simulink model "Pendulum"  (R2024b)
settings: Solver=ode45  StartTime=0.0  StopTime=20  MaxStep=1e-2  RelTol=1e-3  EnableMultiTasking=on
InitFcn:
  | g = 9.81; %gravitational constant
  | 
  | %% S-function
  | % showVR = 0;
  | % CartBlocking = 0;
  | % CartHard = 0;
  | % phi0 = 0; %initial conditions
values from neighbouring files (symbols this model uses):
  A_down = double(subs(A_sym, [X; u], [X_down; u_eq]))    [linearization.m]    (also in my_pendulum.m)
  B_down = double(subs(B_sym, [X; u], [X_down; u_eq]))    [linearization.m]    (also in my_pendulum.m)
  C = [0 1 0 0 ... (first row only)    [linearization.m]    (also in my_pendulum.m)
  D = [0; 0]    [linearization.m]    (also in my_pendulum.m)
  Kp = 10.2    [my_pendulum.m]
libraries: vrlib x4, slpidlib x1
CloseFcn:
  | vrclose all;
  | clear figureVR worldVR;
settings Model: Creator=H  LastModifiedBy=jx2004
settings SolverCC: AlgebraicLoopSolver=TrustRegion
settings DataIOCC: LimitDataPoints=on  SaveFormat=Array  SignalLoggingSaveFormat=ModelDataLogs  ReturnWorkspaceOutputs=off
settings OptimizationCC: ExpressionDepthLimit=2147483647  InitFltsAndDblsToZero=on  LifeSpan=inf
settings DebuggingCC: SaveWithParameterizedLinksMsg=none  UnderspecifiedInitializationDetection=Classic  MergeDetectMultiDrivingBlocksExec=none  SignalResolutionControl=TryResolveAllWithWarning  SolverPrmCheckMsg=warning  FcnCallInpInsideContextMsg=warning  UnconnectedInputMsg=warning  UnconnectedOutputMsg=warning  UnconnectedLineMsg=warning  StateNameClashWarn=warning  SFUnexpectedBacktrackingDiag=warning  SFNoUnconditionalDefaultTransitionDiag=warning  SFExecutionAtInitializationDiag=none  ArithmeticOperatorsInVariantConditions=warning
settings HardwareCC: ProdBitPerPointer=32  ProdBitPerSizeT=32  ProdBitPerPtrDiffT=32  ProdLargestAtomicFloat=None  ProdIntDivRoundTo=Undefined  ProdEndianess=Unspecified  ProdWordSize=32  ProdHWDeviceType=32-bit Generic
settings ModelReferenceCC: PropagateSignalLabelsOutOfModel=off
settings SFSimCC: SimUseLocalCustomCode=off  CustomCodeUndefinedFunction=UseInterfaceOnly
settings RTWCC: RTWUseLocalCustomCode=off  GPUComputeCapability=3.5
settings CodeAppCC: StateflowObjectComments=on
settings GRTTargetCC: TargetFcnLib=ansi_tfl_tmw.mat  TargetLangStandard=C89/C90 (ANSI)  CombineOutputUpdateFcns=off  GRTInterface=on
settings ConfigComp: CovMetricSettings=dw  CovSaveCumulativeToWorkspaceVar=on  CovSaveSingleToWorkspaceVar=on  CovExternalEMLEnable=off

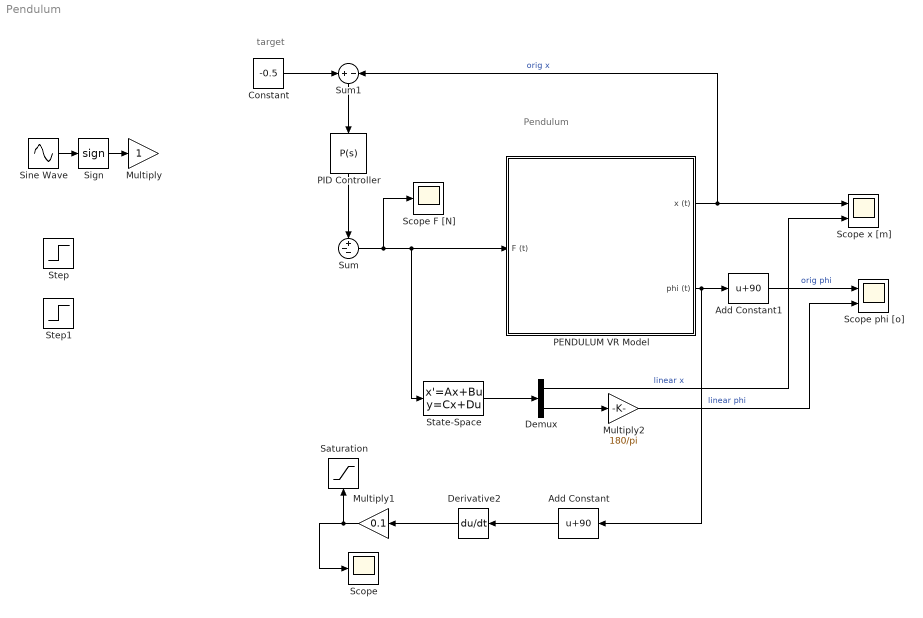
== system Pendulum ==
  note: target
  note: Pendulum
  Add Constant : Bias  Bias=90  SaturateOnIntegerOverflow=off
  Add Constant1 : Bias  Bias=90  SaturateOnIntegerOverflow=off
  Constant : Constant  Value=-0.5
  Demux : Demux  Outputs=2
  Derivative2 : Derivative
  Multiply : Gain
  Multiply1 : Gain  Gain=0.1
  Multiply2 : Gain  Gain=180/pi
  PENDULUM VR Model : Subsystem  mask(Pendulum){showVR=on, phi0=-90, y0=0, brake=off, rail_bound=off}
      mask prompts: showVR "Show Virtual World?"; phi0 "Initial angle of the pendulum   phi(0) [deg] (from horizontal plane)"; y0 "Initial position of the cart x0 [m] (rightwise from the center)"; brake "Cart brake"; rail_bound "Obey rail boundaries"
      mask help: Pendulum - Virtual Reality
      mask init:
      | clear figureVR worldVR;
      | showVR = 1;
      mask Help:
      | Pendulum - Virtual Reality. <br><br>
      | 
      | This is a model of the inverted pendulum on a cart, which consit of a beam and a cart. The beam is connected with the cart by a pivot. The input of this system is mechanical force applied on the cart, outputs are the angle of the beam and the position of the cart.   <br><br>
      | 
      | 
      | In the mask of the model, it can be set:
      | <ul>
      | <li>Initial angle of the pendulum</li>
      | </ul><br><br>
      | 
      | 
      | Copyright: 2007,   Jan Vana, Jirka Roubal, Petr Husek.
      mask Callback showVR:
      | if strcmp('off',get_param(gcb,'showVR'))
      |     vrclose all;
      | else
      |     if exist('figureVR')==0
      |         figureVR = vrfigure;
      |     end
      |     if exist('worldVR')==0
      |         worldVR = vrworld('Pendulum_VR.WRL');
      |     end
      | 	if isvalid(figureVR)==0
      |         open(worldVR);
      |         figureVR = vrfigure(worldVR,[650 80 550 350]);
      | 	end
      | end
      mask Display:
      | image(imread('Pendulum_Image.jpg'))
      | port_label ('input',1,'F')
      | port_label ('output',1,'x')
      | port_label ('output',2,'phi')
  PID Controller : slpidlib/PID Controller  Controller=P  Form=Parallel  TimeDomain=Continuous-time  UseExternalTs=off  SampleTime=-1  IntegratorMethod=Forward Euler  FilterMethod=Forward Euler  ControllerParametersSource=internal  P=Kp  I=1  UseKiTs=off  D=1  UseExternalDerivativeSource=off  N=100  UseFilter=on  TunerSelectOption=Transfer Function Based (PID Tuner App)  InitialConditionSource=internal  InitialConditionForIntegrator=0  InitialConditionForFilter=0  DifferentiatorICPrevScaledInput=0  ExternalReset=none  TrackingMode=off  Kt=1  LimitOutput=off  SatLimitsSource=internal  UpperSaturationLimit=inf  LowerSaturationLimit=-inf  LinearizeAsGain=on  AntiWindupMode=none  Kb=1  LimitIntegrator=off  UpperIntegratorSaturationLimit=inf  LowerIntegratorSaturationLimit=-inf  POutMin=[]  POutMax=[]  IOutMin=[]  IOutMax=[]  DOutMin=[]  DOutMax=[]  NOutMin=[]  NOutMax=[]  SumOutMin=[]  SumOutMax=[]  SaturationOutMin=[]  SaturationOutMax=[]  PParamMin=[]  PParamMax=[]  IParamMin=[]  IParamMax=[]  DParamMin=[]  DParamMax=[]  NParamMin=[]  NParamMax=[]  KbParamMin=[]  KbParamMax=[]  KtParamMin=[]  KtParamMax=[]  KbOutMin=[]  KbOutMax=[]  KtOutMin=[]  KtOutMax=[]  IntegratorOutMin=[]  IntegratorOutMax=[]  FilterOutMin=[]  FilterOutMax=[]  SumI1OutMin=[]  SumI1OutMax=[]  SumI2OutMin=[]  SumI2OutMax=[]  SumI3OutMin=[]  SumI3OutMax=[]  SumI4OutMin=[]  SumI4OutMax=[]  SumDOutMin=[]  SumDOutMax=[]  DifferentiatorOutMin=[]  DifferentiatorOutMax=[]  FilterDiffOutCoefMin=[]  FilterDiffOutCoefMax=[]  ReciprocalOutMin=[]  ReciprocalOutMax=[]  SumDenOutMin=[]  SumDenOutMax=[]  SumNumOutMin=[]  SumNumOutMax=[]  DivideOutMin=[]  DivideOutMax=[]  UdiffTsProdOutMin=[]  UdiffTsProdOutMax=[]  NTsProdOutMin=[]  NTsProdOutMax=[]  UintegralTsProdOutMin=[]  UintegralTsProdOutMax=[]  UngainTsProdOutMin=[]  UngainTsProdOutMax=[]  ClampingZeroOutDataTypeStr=Inherit: Inherit via back propagation  ClampingZeroOutMin=[]  ClampingZeroOutMax=[]  FilterDenConstantOutDataTypeStr=Inherit: Inherit via back propagation  FilterDenConstantOutMin=[]  FilterDenConstantOutMax=[]  PCopyOutDataTypeStr=Inherit: Inherit via back propagation  PCopyOutMin=[]  PCopyOutMax=[]  NCopyOutDataTypeStr=Inherit: Inherit via back propagation  NCopyOutMin=[]  NCopyOutMax=[]  IntegratorContinuousStateAttributes=''  IntegratorStateMustResolveToSignalObject=off  IntegratorRTWStateStorageClass=Auto  FilterContinuousStateAttributes=''  FilterStateMustResolveToSignalObject=off  FilterRTWStateStorageClass=Auto  ParallelPVariant=InternalParameters  IdealPVariant=Disabled  IVariant=Disabled  DVariant=Disabled  IntegratorVariant=Disabled  SatVariant=Disabled  AWVariant=Disabled  PCopyVariant=Disabled  TRVariant=Disabled  FdbkBlocksVariant=Forward  IdealPFdbkVariant=Disabled  SatFdbkVariant=Disabled  DerivativeFilterVariant=Disabled  NVariant=Disabled  NCopyVariant=Disabled_SignalSpec  FilterICVariant=Disabled  IntegratorICVariant=Disabled  ExternalResetVariant=Disabled  TRSumVariant=Passthrough  SumFdbkVariant=Disabled  SumVariant=Passthrough_P  TsampFilterVariant=InternalTs  TsampNgainVariant=Passthrough  TsampIntegralVariant=Disabled_SignalSpec  ExternalSaturationOutDataTypeStr=Inherit: Same as second input  DerivativeSourceVariant=Disabled  PreIntVariant=InternalPreInt
  Saturation : Saturate  UpperLimit=10  LowerLimit=-10  LinearizeAsGain=off  ZeroCross=off
  Scope : Scope
  Scope phi [o] : Scope  NumInputPorts=2
  Scope x [m] : Scope  NumInputPorts=2
  Scope F [N] : Scope
  Sign : Signum
  Sine Wave : Sin  Frequency=1.2  SampleTime=0
  State-Space : StateSpace  A=A_down  B=B_down  C=C  D=D  InitialCondition=[0; 0; 0; 0]
  Step : Step  Time=0  After=5  SampleTime=0
  Step1 : Step  Time=2  After=5  SampleTime=0
  Sum : Sum  Inputs=+--
  Sum1 : Sum  Inputs=+-
  wires:
  Sum/1 -> Scope F [N]/1, State-Space/1, PENDULUM VR Model/1(F (t))
  PENDULUM VR Model/2(phi (t)) -> Add Constant1/1, Add Constant/1
  Sine Wave/1 -> Sign/1
  Sign/1 -> Multiply/1
  Multiply1/1 -> Scope/1, Saturation/1
  Derivative2/1 -> Multiply1/1
  Add Constant/1 -> Derivative2/1
  State-Space/1 -> Demux/1
  Demux/1 -> Scope x [m]/2  "linear x"
  Demux/2 -> Multiply2/1
  Add Constant1/1 -> Scope phi [o]/1  "orig phi"
  Multiply2/1 -> Scope phi [o]/2  "linear phi"
  PENDULUM VR Model/1(x (t)) -> Sum1/2, Scope x [m]/1  "orig x"
  Constant/1 -> Sum1/1
  Sum1/1 -> PID Controller/1
  PID Controller/1 -> Sum/1

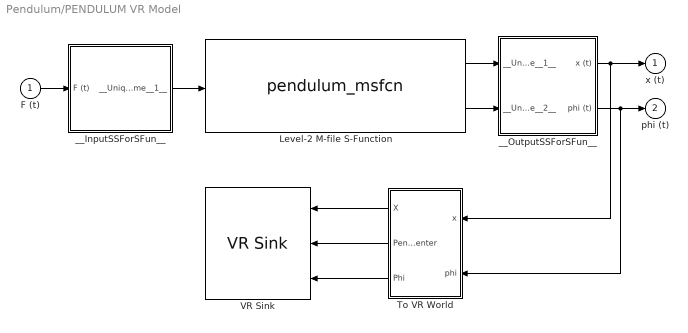
== system Pendulum/PENDULUM VR Model ==
  F (t) : Inport
  Level-2 M-file S-Function : M-S-Function  FunctionName=pendulum_msfcn  Parameters=y0, phi0, rail_bound, brake
  To VR World : Subsystem
  VR Sink : vrlib/VR Sink  InstantiateOnLoad=on  SampleTime=0.1  ViewEnable=on  RemoteChange=off  RemoteView=on  FieldsWritten=cart.translation.3.1.double#pendulum.center.3.1.double#pendulum.rotation.4.1.double  WorldFileName=Pendulum_VR.WRL  AutoView=off  VideoDimensions=[]  AllowVariableSize=off
  __InputSSForSFun__ : Subsystem
  __OutputSSForSFun__ : Subsystem
  x (t) : Outport  OutDataTypeStr=double  PortDimensions=1  SampleTime=[-1 0]
  phi (t) : Outport  Port=2  OutDataTypeStr=double  PortDimensions=1  SampleTime=[-1 0]
  wires:
  To VR World/1(X) -> VR Sink/1
  To VR World/2(Pend center) -> VR Sink/2
  To VR World/3(Phi) -> VR Sink/3
  __OutputSSForSFun__/2(phi (t)) -> To VR World/2(phi), phi (t)/1
  __OutputSSForSFun__/1(x (t)) -> To VR World/1(x), x (t)/1
  Level-2 M-file S-Function/2 -> __OutputSSForSFun__/2(__UniqueInportName__2__)
  Level-2 M-file S-Function/1 -> __OutputSSForSFun__/1(__UniqueInportName__1__)
  __InputSSForSFun__/1(__UniqueOutportName__1__) -> Level-2 M-file S-Function/1
  F (t)/1 -> __InputSSForSFun__/1(F (t))

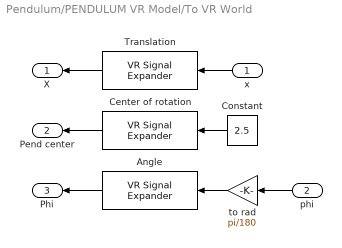
== system Pendulum/PENDULUM VR Model/To VR World ==
  x : Inport
  phi : Inport  Port=2
  Angle : vrlib/VR Signal Expander  outwidth=4  outidx=[4]
  Center of rotation : vrlib/VR Signal Expander  outwidth=3  outidx=[2]
  Constant : Constant  Value=2.5
  Translation : vrlib/VR Signal Expander  outwidth=3  outidx=[1]
  to rad : Gain  Gain=pi/180
  X : Outport
  Pend center : Outport  Port=2
  Phi : Outport  Port=3
  wires:
  Angle/1 -> Phi/1
  Center of rotation/1 -> Pend center/1
  Translation/1 -> X/1
  phi/1 -> to rad/1
  x/1 -> Translation/1
  to rad/1 -> Angle/1
  Constant/1 -> Center of rotation/1

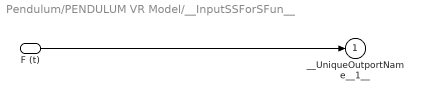
== system Pendulum/PENDULUM VR Model/__InputSSForSFun__ ==
  F (t) : Inport
  __UniqueOutportName__1__ : Outport
  wires:
  F (t)/1 -> __UniqueOutportName__1__/1

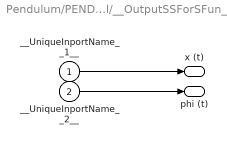
== system Pendulum/PENDULUM VR Model/__OutputSSForSFun__ ==
  __UniqueInportName__1__ : Inport
  __UniqueInportName__2__ : Inport  Port=2
  x (t) : Outport  OutDataTypeStr=double  PortDimensions=1  SampleTime=[-1 0]
  phi (t) : Outport  Port=2  OutDataTypeStr=double  PortDimensions=1  SampleTime=[-1 0]
  wires:
  __UniqueInportName__2__/1 -> phi (t)/1
  __UniqueInportName__1__/1 -> x (t)/1
